simulink model "diag_bloques"  (Simulink 5.0)
settings: Solver=ode45  StartTime=0.0  StopTime=10.0  RelTol=1e-3
libraries: simulink_extras x3
settings Model: LastModifiedBy=pc1

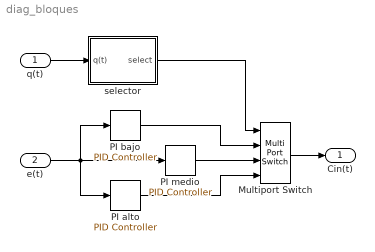
== system diag_bloques ==
  q(t) : Inport
  e(t) : Inport  Port=2
  Multiport Switch : MultiPortSwitch  Inputs=3  SaturateOnIntegerOverflow=on
  PI alto : simulink_extras/Additional Linear/PID Controller  P=.6  I=.6/.8  D=0
  PI bajo : simulink_extras/Additional Linear/PID Controller  P=.12  I=.12/1.1  D=0
  PI medio : simulink_extras/Additional Linear/PID Controller  P=.37  I=.37/1.1  D=0
  selector : Subsystem
  Cin(t) : Outport
  wires:
  e(t)/1 -> PI medio/1, PI bajo/1, PI alto/1
  PI bajo/1 -> Multiport Switch/2
  PI medio/1 -> Multiport Switch/3
  PI alto/1 -> Multiport Switch/4
  Multiport Switch/1 -> Cin(t)/1
  q(t)/1 -> selector/1(q(t))
  selector/1(select) -> Multiport Switch/1

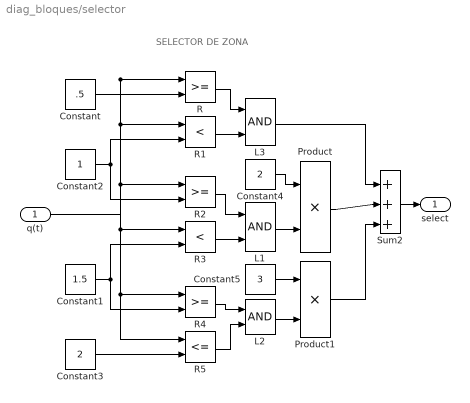
== system diag_bloques/selector ==
  note: SELECTOR DE ZONA
  q(t) : Inport
  Constant : Constant  Value=.5
  Constant1 : Constant  Value=1.5
  Constant2 : Constant
  Constant3 : Constant  Value=2
  Constant4 : Constant  Value=2
  Constant5 : Constant  Value=3
  L1 : Logic  AllPortsSameDT=off
  L2 : Logic  AllPortsSameDT=off
  L3 : Logic  AllPortsSameDT=off
  Product : Product  SaturateOnIntegerOverflow=on
  Product1 : Product  SaturateOnIntegerOverflow=on
  R : RelationalOperator
  R1 : RelationalOperator  Operator=<
  R2 : RelationalOperator
  R3 : RelationalOperator  Operator=<
  R4 : RelationalOperator
  R5 : RelationalOperator  Operator=<=
  Sum2 : Sum  Inputs=|+++  SaturateOnIntegerOverflow=on
  select : Outport
  wires:
  Constant/1 -> R/2
  q(t)/1 -> R/1, R1/1, R2/1, R3/1, R4/1, R5/1
  R/1 -> L3/1
  Constant2/1 -> R1/2, R2/2
  R1/1 -> L3/2
  Constant1/1 -> R3/2, R4/2
  R2/1 -> L1/1
  R3/1 -> L1/2
  Constant3/1 -> R5/2
  R5/1 -> L2/2
  Constant4/1 -> Product/1
  L1/1 -> Product/2
  Constant5/1 -> Product1/1
  L2/1 -> Product1/2
  L3/1 -> Sum2/1
  Product/1 -> Sum2/2
  Product1/1 -> Sum2/3
  Sum2/1 -> select/1
  R4/1 -> L2/1
